simulink model "VFlexP"  (R2025a)
settings: Solver=ode23tb  StartTime=0.0  StopTime=40  FixedStep=5e-5
model workspace (MAT data in the model file):
  DCop_DCBUCK : object (value not decoded)
  Grid_CCVSC_idx = [2; 3; 4; 5; 6; 7; 8; 9; 10; 11; 12]
  Grid_CCVSCs = 1
  Grid_CCVSCs_buses = 1
  Grid_CCVSCs_toM = [0 1 0 0 0 0 0 0 0 0 0 0 ... (781 elements, 71x11)]
  Grid_C_Lines = [0.1 0.1 0.1 0.1]
  Grid_Cbuses = [0.05000002 0.10000002 0.10000002 0.10000002 0.05000002]
  Grid_DC : object (value not decoded)
  Grid_DCop_DCBUCK : object (value not decoded)
  Grid_DCop_DC_PES : object (value not decoded)
  Grid_DFIGs = 1
  Grid_DFIGs_buses = 1
  Grid_DGs : string (value not decoded)
  Grid_From_buses = [1 2 4 4]
  Grid_GFls = 1
  Grid_GFls_buses = 1
  Grid_GFr_idx = [1; 2; 3]
  Grid_GFrs = 1
  Grid_GFrs_buses = 1
  Grid_GFrs_toM = [1 0 0 0 0 0 0 0 0 1 0 0 ... (15 elements, 5x3)]
  Grid_IG_idx = 1
  Grid_IGs = 1
  Grid_IGs_buses = 1
  Grid_IGs_toM = [1; 0]
  Grid_L_Lines = [0.5 0.5 0.5 0.5]
  Grid_L_Loads = [0.000959999944704 0.000156249997559 0.00154855477548]
  Grid_Lines_fromM : object (value not decoded)
  Grid_Lines_toM : object (value not decoded)
  Grid_Load_buses = [2; 3; 4]
  Grid_Load_busesDC = []
  Grid_MGES_idx = [1; 2; 3]
  Grid_MGESs = 1
  Grid_MGESs_buses = [1; 5; 3]
  Grid_MGESs_toM = [1 0 0 0 0 0 0 0 0 1 0 0 ... (15 elements, 5x3)]
  Grid_MSGs = 1
  Grid_MSGs_buses = 1
  Grid_Nbuses = 5
  Grid_PQ_gen = [3; 2; 2]
  Grid_Ploads = [1250 4000 1250]
  Grid_PloadsDC = []
  Grid_Ps_lf = [0.274439537683 0.78 0.3]
  Grid_Qloads = [0.3 0.5 0.5]
  Grid_Qs_lf = [-0.0366071562958 0.126505596722 -0.0162964024532]
  Grid_R_Lines = [0.01 0.01 0.01 0.01]
  Grid_R_Loads = [3.9999997696 1.24999998047 3.8713869387]
  Grid_R_Loads_DC = 0
  Grid_Rcf = [50000000 50000000 50000000 50000000 50000000]
  Grid_SCs = 1
  Grid_SCs_buses = 1
  Grid_SG_idx = 1
  Grid_SGs = 1
  Grid_SGs_buses = 1
  Grid_SGs_toM = [1; 0]
  Grid_To_buses = [2 3 3 5]
  Grid_VCVSC_idx = [1; 2; 3; 4; 5; 6; 7; 8; 9; 10; 11; 12]
  Grid_VCVSCs = 1
  Grid_VCVSCs_buses = [1; 2; 3; 6; 8; 9; 12; 58; 59; 60; 63; 65]
  Grid_VCVSCs_toM = [1 0 0 0 0 0 0 0 0 0 0 0 ... (852 elements, 71x12)]
  Grid_VSM_idx = [1; 2; 3]
  Grid_VSMs = 1
  Grid_VSMs_buses = 1
  Grid_VSMs_toM = [1 0 0 0 0 0 0 0 0 1 0 0 ... (15 elements, 5x3)]
  Grid_admitt_matrix = [2.15353135314-19.7953135314i  -1.9801980198+19.801980198i; -1.9801980198+19.801980198i  2.15353135314-19.7953135314i]
  Grid_admitt_matrix_noloads = [1.98686468647-19.7953135314i  -1.9801980198+19.801980198i; -1.9801980198+19.801980198i  1.98686468647-19.7953135314i]
  Grid_bus = [1; 2; 6; 7; 8]
  Grid_busDC_complexity = [1 1 1]
  Grid_busDC_complexity_PF = [2 2 2]
  Grid_bus_complexity = [1 1 1 1 1]
  Grid_bus_complexity_PF = [1 1 1 1 1]
  Grid_buses_lf = [1; 5; 3]
  Grid_conductance_matrix = [100.00000002  -100  0; -100  200.00000002  -100; 0  -100  100.00000002]
  Grid_conductance_matrix_noloads = [100.00000002  -100  0; -100  200.00000002  -100; 0  -100  100.00000002]
  Grid_fref : object (value not decoded)
  Grid_gen_static_params : mBase (value not decoded)
  Grid_iPs_lf = [3.64378984326 1.28205128205 3.33333333333]
  Grid_iQs_lf = [-27.3170631425 7.90478860943 -61.3632366329]
  Grid_iadmitt_matrix = [2.88165849328-0.0982918688642i  2.87905051706-0.123273862303i; 2.87905051706-0.123273862303i  2.88165849328-0.0982918688642i]
  Grid_iadmitt_matrix_noloads = [37.5012524798-37.4874983544i  37.4987475202-37.5125016456i; 37.4987475202-37.5125016456i  37.5012524798-37.4874983544i]
  Grid_iconductance_matrix = [16666671.4556  16666671.4489  16666671.4456; 16666671.4489  16666671.4522  16666671.4489; 16666671.4456  16666671.4489  16666671.4556]
  Grid_iconductance_matrix_noloads = [16666671.4556  16666671.4489  16666671.4456; 16666671.4489  16666671.4522  16666671.4489; 16666671.4456  16666671.4489  16666671.4556]
  Grid_init_OK_bool = 1
  Grid_intconv_PF : object (value not decoded)
  Grid_lf_op : op_report (value not decoded)
  Grid_lineDC_complexity = [1 1]
  Grid_lineDC_complexity_PF = [2 2]
  Grid_line_complexity = [1 1 1 1]
  Grid_line_complexity_PF = [3 3 3 3]
  Grid_loadDC_complexity = []
  Grid_loadDC_complexity_PF = []
  Grid_load_complexity = [3 3 3]
  Grid_load_complexity_PF = [4 4 4]
  Grid_opDC_CCVSC : object (value not decoded)
  Grid_opDC_VSM : object (value not decoded)
  Grid_opGFr : object (value not decoded)
  Grid_opVCVSC : object (value not decoded)
  Grid_op_CCVSC : object (value not decoded)
  Grid_op_IG : object (value not decoded)
  Grid_op_MGES : object (value not decoded)
  Grid_op_SG : object (value not decoded)
  Grid_op_VSM : object (value not decoded)
  Grid_shift_lines = [0 0 0 0]
  Grid_tap_lines = [1 1 1 1]
  Grid_v_buses_mod = [1 1 1 0.9837920967 1]
  LinsysParamChangeStruct : Param1 (value not decoded)
  Lline = 0.01
  Rline = 1e-05
  linsys : object (value not decoded)
symbols that are objects in the model workspace (value not decoded): Grid_DCop_DC_PES, Grid_DCop_DCBUCK, Grid_op_CCVSC, Grid_op_IG, Grid_op_MGES, Grid_op_SG, Grid_op_VSM, Grid_opDC_CCVSC, Grid_opDC_VSM, Grid_opGFr, Grid_opVCVSC
undefined symbols (not defined in the file): block_buses_DC, block_idx, CCVSC_idx, Cf, costs, costs2, D, DFIGs_nodes, DiscIntNeverNeededParam, entity, Fb, Fi, From_nodes, grid_linsys, Grid_op_DFIG, Grid_op_DFIG_PQ, Grid_op_MSG, Grid_op_SC, Grid_op_VCVSC, H, initial_states_grid, K_1, K_3, K_5, K_A, K_C, K_IM, K_IR, K_P, K_PM, K_PR, K_S1, K_S2, K_S3, Ki_w, Kic, Kiv, Kp_id, Kp_theta, Kp_w, Kpc, Kpv, last_send, Lc, Lf, Lfd, Lkd1, Lkd2, Lkq1, Lkq2, Lkq3, Lmd, Lmq, Lsd, Lsq, m, M, Matrix_flux_to_i, mp, MSGs_buses ... (+44)
libraries: simulink x1048, eeGeneralControl x12
(part 7 of 50)

== system VFlexP/Grid/Generators/VSM ==
  note: port number 2
  note: do not rename this block, conditions to initialise the generator from PF result are set on this block's output
  note: port number 1
  elec_in : Inport
  v : Inport  Port=2
  AND : Logic  IconShape=distinctive  AllPortsSameDT=off  OutDataTypeStr=boolean
  AND1 : Logic  Inputs=3  IconShape=distinctive  AllPortsSameDT=off  OutDataTypeStr=boolean
  AND2 : Logic  IconShape=distinctive  AllPortsSameDT=off  OutDataTypeStr=boolean
  Abs{,1..3} (4 alike) : Abs  ZeroCross=off  SaturateOnIntegerOverflow=off
  Assignment : Assignment  NumberOfDimensions=2  DiagnosticForDimensions=Warning  IndexOptions=Assign all,Index vector (dialog)  Indices=1,block_idx  OutputSizes=1,1
  Atan2 : Trigonometry  Operator=atan2
  Cast To Boolean : DataTypeConversion  OutDataTypeStr=boolean  SaturateOnIntegerOverflow=off  RndMeth=Floor
  Cast To Double : DataTypeConversion  OutDataTypeStr=double  SaturateOnIntegerOverflow=off  RndMeth=Floor
  Cast To Double1 : DataTypeConversion  OutDataTypeStr=double  SaturateOnIntegerOverflow=off  RndMeth=Floor
  Cast To Double2 : DataTypeConversion  OutDataTypeStr=double  SaturateOnIntegerOverflow=off  RndMeth=Floor
  Compare To Constant : simulink/Logic and Bit Operations/Compare To Constant  relop=<=  const=0.001  OutDataTypeStr=boolean  ZeroCross=off
  Compare To Constant1 : simulink/Logic and Bit Operations/Compare To Constant  relop=<=  const=0.01  OutDataTypeStr=boolean  ZeroCross=off
  Compare To Constant2 : simulink/Logic and Bit Operations/Compare To Constant  relop=<=  const=0.2  OutDataTypeStr=boolean  ZeroCross=off
  Compare To Constant3 : simulink/Logic and Bit Operations/Compare To Constant  relop=>  const=4  OutDataTypeStr=boolean  ZeroCross=off
  Complex to Magnitude-Angle1 : ComplexToMagnitudeAngle  Output=Magnitude
  Complex to Real-Imag : ComplexToRealImag
  Conjugate : Math  Operator=conj  SignedPower=on  RndMeth=Zero
  Constant : Constant  Value=zeros(1, length(block_buses))  VectorParams1D=off
  Constant1 : Constant  Value=5*ones(1,length(block_idx))  VectorParams1D=off
  Constant2 : Constant  Value=zeros(1,length(block_idx))  VectorParams1D=off
  For Each Subsystem : Subsystem  TreatAsAtomicUnit=on
  Gain1 : Gain  Gain=-1
  Gain2 : Gain  Gain=-1
  Integrator : Integrator  ExternalReset=falling  InitialConditionSource=external  InitialCondition=[5]
  LPF1 : Subsystem
  LPF4 : Subsystem  Commented=through
  LPF5 : Subsystem  Commented=through
  Matrix Concatenate : Concatenate  NumInputs=6  Mode=Multidimensional array
  Matrix Concatenate1 : Concatenate  NumInputs=3  Mode=Multidimensional array
  Memory : Memory  InitialCondition=1
  Memory1 : Memory  InitialCondition=1
  Memory2 : Memory  InitialCondition=1
  NOT1 : Logic  Operator=NOT  IconShape=distinctive  AllPortsSameDT=off  OutDataTypeStr=boolean
  OR : Logic  Operator=OR  Inputs=3  IconShape=distinctive  AllPortsSameDT=off  OutDataTypeStr=boolean
  PC : Subsystem  mask(PC_VCVSC){Tf=Tf/(2*mp), mp=mp, nq=nq}
      mask prompts: Tf "Low-pass filter time constant (s)"; mp "Droop coefficient mp"; nq "Droop coefficient nq"
      mask help: Power controller of a grid-forming converter, including the droop control and low-pass filters for the power measurements.
      mask init: same as VFlexP/Grid/DCAC converters/DC_VCVSC/PC
  PI : Subsystem  Commented=on
  PI1 : Subsystem  Commented=on
  Product : Product
  Product1 : Product  OutDataTypeStr=double
  Product2 : Product  OutDataTypeStr=double
  Product3 : Product
  RL out : Subsystem  Variant=on  VariantControlMode=label  LabelModeActiveChoice=dynamic  mask{dynamic=Dynamic, R=R_out, L=L_out, fbase=50}
      mask prompts: dynamic "Dynamic behavior"; R "Series resistance (p.u.)"; L "Inductance (p.u.)"; fbase "Base frequency (Hz)"
      mask init: same as VFlexP/Grid/DCAC converters/DC_VCVSC/RL out
      mask TypeOptions dynamic: Static | Dynamic | Static omega
  Rate Limiter : RateLimiter  Commented=through  RisingSlewLimit=0.01  FallingSlewLimit=-0.01  SampleTimeMode=inherited
  Rate Limiter1 : RateLimiter  Commented=through  RisingSlewLimit=0.01  FallingSlewLimit=-0.01  SampleTimeMode=inherited
  Real-Imag to Complex : RealImagToComplex
  Real-Imag to Complex1 : RealImagToComplex
  Real-Imag to Complex3 : RealImagToComplex
  Reference frame transform1 : Subsystem
  Reference frame transform2 : Subsystem
  Reference frame transform3 : Subsystem
  Selector : Selector  NumberOfDimensions=2  InputPortWidth=3  IndexOptions=Index vector (dialog),Index vector (dialog)  Indices=1,block_idx  OutputSizes=1,1
  Selector1 : Selector  NumberOfDimensions=2  InputPortWidth=3  IndexOptions=Index vector (dialog),Index vector (dialog)  Indices=2,block_idx  OutputSizes=1,1
  Selector2 : Selector  NumberOfDimensions=2  InputPortWidth=3  IndexOptions=Index vector (dialog),Index vector (dialog)  Indices=3,block_idx  OutputSizes=1,1
  Selector3 : Selector  NumberOfDimensions=2  InputPortWidth=3  IndexOptions=Index vector (dialog),Index vector (dialog)  Indices=4,block_idx  OutputSizes=1,1
  Selector4 : Selector  NumberOfDimensions=2  InputPortWidth=3  IndexOptions=Index vector (dialog),Index vector (dialog)  Indices=5,block_idx  OutputSizes=1,1
  Selector5 : Selector  NumberOfDimensions=2  InputPortWidth=3  IndexOptions=Index vector (dialog),Index vector (dialog)  Indices=1,block_buses  OutputSizes=1,1
  Selector6 : Selector  NumberOfDimensions=2  InputPortWidth=3  IndexOptions=Index vector (dialog),Index vector (dialog)  Indices=2,block_buses  OutputSizes=1,1
  Selector7 : Selector  InputPortWidth=length(fref.ref_units)  IndexOptions=Index vector (dialog)  Indices=block_fref  OutputSizes=1
  Selector8 : Selector  InputPortWidth=length(fref.ref_units)  IndexOptions=Index vector (dialog)  Indices=block_fref  OutputSizes=1
  Signal Specification : SignalSpecification  Dimensions=[6 length(buses_lf)]
  Signal Specification1 : SignalSpecification  Dimensions=[3 length(block_buses)]
  Step : Step  Time=0.01  SampleTime=0  VectorParams1D=off  ZeroCross=off
  Sum10 : Sum  Inputs=|++
  Sum2 : Sum  Inputs=-+|
  Sum3 : Sum  Inputs=|+-
  Sum8 : Sum  Inputs=++|
  Sum9 : Sum  Inputs=|++
  Switch : Switch  Criteria=u2 > Threshold  SaturateOnIntegerOverflow=off  InputSameDT=off
  Switch1 : Switch  Criteria=u2 > Threshold  SaturateOnIntegerOverflow=off  InputSameDT=off
  Switch2 : Switch  Criteria=u2 > Threshold  SaturateOnIntegerOverflow=off  InputSameDT=off
  Terminator{,1..5} (6 alike) : Terminator
  VCC : Subsystem  Variant=on  VariantControlMode=label  LabelModeActiveChoice=static
  VI : Subsystem  mask{L=VI_L, R=VI_R, Tf=WOF_Tf}
      mask prompts: L "Inductance (pu)"; R "Resistance (pu)"; Tf "WOF time constant (s)"
      mask init: same as VFlexP/Grid/DCAC converters/DC_VCVSC/VI
  Zero : Constant  Value=0  OutDataTypeStr=Inherit: Inherit via back propagation
  Zero1 : Constant  Value=zeros(6, length(buses_lf))  VectorParams1D=off  OutDataTypeStr=Inherit: Inherit via back propagation
  connect : Subsystem
  frame : Integrator  InitialCondition=Grid_op_VSM.op.States(17).x'  IgnoreLimit=on
  trim_output : Subsystem
  vod : Sum  Inputs=++|
  elec_out : Outport
  i : Outport  Port=2
  wires:
  VCC/2(viqref) -> Reference frame transform3/3(in_q), [voq]
  VCC/1(vidref) -> Reference frame transform3/1(in_d), [vod]
  Memory1/1 -> Cast To Boolean/1
  Switch/1 -> Integrator/3
  Cast To Double2/1 -> Integrator/1
  AND1/1 -> Integrator/2, Cast To Double2/1
  [safe_to_connect] -> AND1/3
  Constant1/1 -> Switch/3
  Step/1 -> AND1/1, Switch/2
  Constant2/1 -> Switch/1
  Integrator/1 -> Compare To Constant3/1
  [connect] -> AND1/2
  AND2/1 -> Product2/1, Product1/1
  [connect] -> AND2/2
  [connected] -> NOT1/1
  NOT1/1 -> AND2/1
  [omega_to_follow] -> Sum10/2, Switch2/1
  Selector1/1 -> [P_s_to_follow]
  Memory/1 -> Cast To Double/1
  Selector5/1 -> trim_output/3(vd), [vdout]
  Selector6/1 -> trim_output/4(vq), [vqout]
  v/1 -> Selector5/1, Selector6/1
  trim_output/4(Out4) -> Terminator5/1
  trim_output/3(Out3) -> Terminator4/1
  trim_output/2(Out2) -> Terminator3/1
  trim_output/1(Out1) -> Terminator/1
  Zero1/1 -> Assignment/1
  [v_d_PCC] -> Real-Imag to Complex3/1
  [v_q_PCC] -> Real-Imag to Complex3/2
  Real-Imag to Complex3/1 -> Complex to Magnitude-Angle1/1
  [v_q_PCC] -> PC/5(voq)
  [v_d_PCC] -> PC/4(vodi)
  Signal Specification1/1 -> For Each Subsystem/1(In1)
  For Each Subsystem/1(Out1) -> i/1
  Constant/1 -> Matrix Concatenate1/3
  Matrix Concatenate1/1 -> Signal Specification1/1
  [vdout] -> Reference frame transform2/1(in_d), RL out/2(v_out_d)
  Reference frame transform2/2(out_q) -> [v_q_PCC]
  Reference frame transform2/1(out_d) -> [v_d_PCC]
  [vqout] -> RL out/4(v_out_q), Reference frame transform2/3(in_q)
  Memory2/1 -> [safe_to_connect]
  [connected] -> OR/3
  Compare To Constant2/1 -> OR/2
  OR/1 -> Memory2/1
  AND/1 -> OR/1
  Compare To Constant1/1 -> AND/1
  Abs3/1 -> Compare To Constant1/1
  Compare To Constant/1 -> AND/2
  Abs2/1 -> Compare To Constant/1
  Signal Specification/1 -> elec_out/1
  Abs1/1 -> Sum3/2, Compare To Constant2/1
  Cast To Boolean/1 -> [connect]
  Switch2/1 -> Rate Limiter/1
  PI1/1(Out1) -> Sum10/1
  Atan2/1 -> Product2/2, Abs3/1
  Product2/1 -> PI1/1(In1)
  Product1/1 -> PI/1(In1)
  PI/1(Out1) -> Sum9/1
  Sum3/1 -> Product1/2, Abs2/1
  Abs/1 -> Sum3/1
  Complex to Real-Imag/1 -> Atan2/2
  Complex to Real-Imag/2 -> Atan2/1
  Product/1 -> Complex to Real-Imag/1
  Conjugate/1 -> Product/2
  Real-Imag to Complex/1 -> Product/1, Abs/1
  Real-Imag to Complex1/1 -> Conjugate/1, Abs1/1
  [voq] -> Real-Imag to Complex1/2
  [vod] -> Real-Imag to Complex1/1
  [v_q_PCC] -> Real-Imag to Complex/2
  [v_d_PCC] -> Real-Imag to Complex/1
  Cast To Double1/1 -> Matrix Concatenate/5
  Cast To Double/1 -> Matrix Concatenate/6
  Selector4/1 -> Memory1/1
  [connected] -> Memory/1
  [connect] -> Cast To Double1/1
  Assignment/1 -> Signal Specification/1
  elec_in/1 -> Selector/1, Selector1/1, Selector2/1, Selector3/1, Selector4/1
  Matrix Concatenate/1 -> Assignment/2
  [omega] -> Matrix Concatenate/1  "omega"
  Complex to Magnitude-Angle1/1 -> LPF1/1(In1)  "v"
  [P_s] -> Matrix Concatenate/2  "P_s"
  [Q_s] -> Matrix Concatenate/4
  Selector2/1 -> [v_to_follow]
  Selector/1 -> [omega_to_follow]
  Selector3/1 -> [Q_s_to_follow]
  RL out/4(v_outq) -> Terminator2/1
  RL out/3(v_outd) -> Terminator1/1
  connect/2(iq_real) -> Reference frame transform1/3(in_q), Matrix Concatenate1/2, trim_output/2(iq)
  connect/1(id_real) -> Reference frame transform1/1(in_d), Matrix Concatenate1/1, trim_output/1(id)
  VI/2(vq) -> Sum8/1
  VI/1(vd) -> vod/1
  Reference frame transform1/1(out_d) -> [iod]
  RL out/2(iq) -> connect/2(iq)
  Reference frame transform3/2(out_q) -> RL out/3(v_in_q)
  Reference frame transform3/1(out_d) -> RL out/1(v_in_d)
  Reference frame transform1/2(out_q) -> [ioq]
  [ioq] -> PC/1(ioq)
  [iod] -> PC/2(iodi)
  PC/2(Out2) -> [vodref]
  PC/1(omega) -> [omega]
  [theta] -> Reference frame transform3/2(theta)
  [omega] -> VCC/5(omega)
  [vodref] -> vod/2
  Zero/1 -> Sum8/2
  [iod] -> VCC/3(iod)
  [ioq] -> VCC/4(ioq)
  Gain1/1 -> Reference frame transform1/2(theta)
  [theta] -> Gain1/1
  RL out/1(id) -> connect/1(id)
  Sum2/1 -> Product3/1
  [omega_ref] -> Selector7/1  "ref_omega"
  [omega] -> Sum2/2  "omega"
  connect/3(connected) -> [connected]
  PC/3(P_f) -> [P_f], [P_s]
  PC/4(Q_f) -> [Q_f], [Q_s]
  [P_s_to_follow] -> PC/7(Psp)
  frame/1 -> [theta]
  Product3/1 -> frame/1
  Rate Limiter1/1 -> LPF5/1(In1)
  [theta] -> Gain2/1
  Gain2/1 -> Reference frame transform2/2(theta)
  [iod] -> VI/1(id)
  [ioq] -> VI/2(iq)
  [omega] -> VI/3(omega)
  vod/1 -> VCC/1(vodref)
  Sum8/1 -> VCC/2(voqref)
  Rate Limiter/1 -> LPF4/1(In1)
  Sum10/1 -> Switch2/3
  Sum9/1 -> Switch1/3
  [connected] -> Switch1/2, Switch2/2
  Switch1/1 -> Rate Limiter1/1
  [v_to_follow] -> Sum9/2, Switch1/1
  LPF4/1(Out1) -> PC/6(omegasp)
  LPF5/1(Out1) -> PC/3(Eref)
  Selector7/1 -> Sum2/1
  [omega_base] -> Selector8/1
  Selector8/1 -> Product3/2
  LPF1/1(Out1) -> Matrix Concatenate/3
  Compare To Constant3/1 -> connect/3(connect)

== system VFlexP/Grid/Generators_DC/DCBUCK ==
  v : Inport
  ref : Inport  Port=2
  Constant2 : Constant  Value=block_Pg./(DC.v(block_buses)*Sb)  VectorParams1D=off
  Gain : Gain  Gain=0.6
  Gain1 : Gain  Gain=565.4867
  Gain4 : Gain  Gain=1/1.5915e-04
  Gain5 : Gain  Gain=0.01
  Integrator : Integrator  InitialCondition=Grid_DCop_DCBUCK.op.States(1).x'
  Integrator1 : Integrator  InitialCondition=Grid_DCop_DCBUCK.op.States(2).x'
  Selector : Selector  InputPortWidth=DC.Nbuses  IndexOptions=Index vector (dialog)  Indices=block_buses  OutputSizes=1
  Selector1 : Selector  Commented=on  InputPortWidth=3  IndexOptions=Index vector (dialog)  Indices=[1 3]  OutputSizes=1
  State-Space : StateSpace  A=[]  B=[]  C=[]  D=block_toM  InitialCondition=0  ParameterTunability=Optimized
  Sum : Sum  Inputs=|++
  Sum2 : Sum  Inputs=|+-
  Sum3 : Sum  Inputs=++-
  Transpose : Math  Operator=transpose
  Transpose1 : Math  Operator=transpose
  i : Outport
  wires:
  Gain5/1 -> Sum3/3
  Selector/1 -> Sum3/1
  v/1 -> Selector/1
  ref/1 -> Selector1/1
  Constant2/1 -> Sum2/1
  Sum3/1 -> Gain4/1
  Transpose1/1 -> i/1
  Sum2/1 -> Gain/1, Gain1/1
  Gain4/1 -> Integrator/1
  Integrator1/1 -> Sum/1
  Gain/1 -> Sum/2
  Sum/1 -> Sum3/2
  Gain1/1 -> Integrator1/1
  Transpose/1 -> State-Space/1
  Integrator/1 -> Transpose/1, Gain5/1, Sum2/2
  State-Space/1 -> Transpose1/1

== system VFlexP/Grid/Generators_DC/DC_PES ==
  v : Inport
  ref : Inport  Port=2
  Gain : Gain
  Gain1 : Gain  Gain=5.4131
  Gain2 : Gain  Gain=0.0018
  Gain3 : Gain  Gain=5.0000
  Integrator : Integrator  InitialCondition=Grid_DCop_DC_PES.op.States(1).x'
  Integrator1 : Integrator  InitialCondition=Grid_DCop_DC_PES.op.States(2).x'
  Integrator2 : Integrator  InitialCondition=Grid_DCop_DC_PES.op.States(3).x'
  One : Constant  Value=DC.v(block_buses)  OutDataTypeStr=Inherit: Inherit via back propagation
  Selector : Selector  InputPortWidth=DC.Nbuses  IndexOptions=Index vector (dialog)  Indices=block_buses  OutputSizes=1
  Selector1 : Selector  Commented=on  InputPortWidth=3  IndexOptions=Index vector (dialog)  Indices=[1 3]  OutputSizes=1
  Square : Math  Operator=square
  State-Space : StateSpace  A=[]  B=[]  C=[]  D=block_toM  InitialCondition=0  ParameterTunability=Optimized
  Step2 : Step  Time=0.1  After=0.1  SampleTime=0
  Sum : Sum  Inputs=+|+|+
  Sum1 : Sum  Inputs=|+-
  Sum13 : Sum  Inputs=|++
  Sum2 : Sum  Inputs=|+-
  Sum3 : Sum  Inputs=|+-
  Transpose : Math  Operator=transpose
  Transpose1 : Math  Operator=transpose
  WOF_d : Subsystem
  i : Outport
  wires:
  State-Space/1 -> Transpose1/1
  Transpose/1 -> State-Space/1
  Transpose1/1 -> i/1
  Sum3/1 -> Gain2/1, Gain1/1, Gain3/1
  ref/1 -> Selector1/1
  v/1 -> Selector/1
  Selector/1 -> Square/1
  One/1 -> Sum3/1
  Sum1/1 -> Gain/1
  Integrator1/1 -> Sum1/2, Transpose/1
  Gain/1 -> Integrator1/1
  Sum2/1 -> Sum1/1
  Gain2/1 -> WOF_d/1(In1)
  Sum13/1 -> Sum2/1
  Integrator2/1 -> Sum13/2
  Sum/1 -> Sum13/1
  Gain3/1 -> Integrator/1
  Square/1 -> Sum3/2
  Gain1/1 -> Sum/1
  Integrator/1 -> Sum/3
  WOF_d/1(Out1) -> Sum/2

== system VFlexP/Grid/Grid/Dynamic ==
  i_from_gen : Inport
  Buses : Subsystem
  Goto Tag Visibility : GotoTagVisibility  GotoTag=Cbuses
  Lines : Subsystem
  Lines to buses : Subsystem
  Loads : Subsystem
  Loads to buses : Subsystem
  Selector2 : Selector  NumberOfDimensions=2  InputPortWidth=Nnodes  IndexOptions=Select all,Index vector (dialog)  Indices=1,Load_buses  OutputSizes=1,1
  Selector4 : Selector  NumberOfDimensions=2  InputPortWidth=Nnodes  IndexOptions=Select all,Index vector (dialog)  Indices=From_nodes,From_buses  OutputSizes=1,1
  Selector6 : Selector  NumberOfDimensions=2  InputPortWidth=Nnodes  IndexOptions=Select all,Index vector (dialog)  Indices=To_nodes,To_buses  OutputSizes=1,1
  Step : Step  Before=ones(1, length(From_buses))  After=[1 ones(1, length(From_buses)-1)]  SampleTime=0
  Sum : Sum  Inputs=++|
  Sum1 : Sum  Inputs=|++
  connect : Subsystem
  iCbuses : Subsystem
  iP : Subsystem
  v_buses : Outport
  tag scope: Cbuses=scoped
  wires:
  Buses/1(v) -> [v_buses], v_buses/1  "v"
  [i_from_lines] -> Sum/2
  [i_to_loads] -> Sum1/1
  Lines to buses/2(i_out_buses) -> [i_to_lines]
  Loads to buses/1(i_out_buses) -> [i_to_loads]
  iP/1(Out1) -> Loads/3(iP)
  Selector6/1 -> Lines/2(v_out)
  [v_buses] -> Selector2/1
  connect/1(Out1) -> Loads/2(connected)
  [v_buses] -> Selector6/1
  Loads/1(i) -> Loads to buses/1(i_loads)
  Sum/1 -> Buses/1(i_in)
  Selector4/1 -> Lines/1(v_in)
  Selector2/1 -> Loads/1(v_in)
  [v_buses] -> Selector4/1
  [i_to_lines] -> Sum1/2
  Step/1 -> iCbuses/1(In1), Lines/3(connected)
  i_from_gen/1 -> Sum/1
  Sum1/1 -> Buses/2(i_out)
  Lines to buses/1(i_in_buses) -> [i_from_lines]
  Lines/1(i) -> Lines to buses/1(i)
  iCbuses/1(Out1) -> [Cbuses]

== system VFlexP/Grid/Grid/Static ==
  i_from_gen : Inport
  Complex to Real-Imag : ComplexToRealImag
  Constant : Constant  Value=zeros(1, Nbuses)  VectorParams1D=off
  Gain : Gain  Gain=iadmitt_matrix  Multiplication=Matrix(K*u)
  Matrix Concatenate : Concatenate  NumInputs=3  Mode=Multidimensional array
  Real-Imag to Complex : RealImagToComplex
  Scope : Scope
      settings: ActiveDisplayYMinimum=1.0463  ActiveDisplayYMaximum=1.1306
  Selector : Selector  NumberOfDimensions=2  InputPortWidth=3  IndexOptions=Index vector (dialog),Select all  Indices=1,find(bus_complexity == 1)  OutputSizes=1,1
  Selector1 : Selector  NumberOfDimensions=2  InputPortWidth=3  IndexOptions=Index vector (dialog),Select all  Indices=2,find(bus_complexity == 1)  OutputSizes=1,1
  Transpose : Math  Operator=transpose
  Transpose2 : Math  Operator=transpose
  v_buses : Outport
  wires:
  Constant/1 -> Matrix Concatenate/3
  Selector/1 -> Real-Imag to Complex/1  "id1"
  Selector1/1 -> Real-Imag to Complex/2  "iq1"
  i_from_gen/1 -> Selector1/1, Selector/1
  Real-Imag to Complex/1 -> Transpose/1
  Complex to Real-Imag/1 -> Matrix Concatenate/1, Scope/1
  Complex to Real-Imag/2 -> Matrix Concatenate/2
  Transpose2/1 -> Complex to Real-Imag/1
  Transpose/1 -> Gain/1
  Gain/1 -> Transpose2/1
  Matrix Concatenate/1 -> v_buses/1

== system VFlexP/Grid/Grid_DC/dynamic ==
  i_from_gen_dc : Inport
  BusesDC : Subsystem
  DC_Lines_toM1 : Subsystem  TreatAsAtomicUnit=on
  DClines : Subsystem
  Loads : Subsystem  Commented=on
  Loads to buses : Subsystem  Commented=on
  One1 : Constant  Commented=on  Value=ones(1, length(R_Loads_DC))  VectorParams1D=off  OutDataTypeStr=Inherit: Inherit via back propagation
  Scope : Scope
      settings: ActiveDisplayYMinimum=-0.01246  ActiveDisplayYMaximum=0.11218
  Selector2 : Selector  NumberOfDimensions=2  InputPortWidth=Nnodes  IndexOptions=Select all,Index vector (dialog)  Indices=From_nodes,DC.to  OutputSizes=1,1
  Selector4 : Selector  NumberOfDimensions=2  InputPortWidth=Nnodes  IndexOptions=Select all,Index vector (dialog)  Indices=From_nodes,DC.from  OutputSizes=1,1
  Selector5 : Selector  Commented=on  NumberOfDimensions=2  InputPortWidth=Nnodes  IndexOptions=Select all,Index vector (dialog)  Indices=1,Load_busesDC  OutputSizes=1,1
  Step1 : Step  Commented=on  Time=1.2  Before=zeros(1, DC.Nbuses)  After=[-0.01 zeros(1, DC.Nbuses-1)]  SampleTime=0  VectorParams1D=off
  Step3 : Step  Commented=on  Before=zeros(1, DC.Nbuses)  After=[0.01 zeros(1, DC.Nbuses-1)]  SampleTime=0  VectorParams1D=off
  Sum : Sum  Commented=on  Inputs=|++
  Sum6 : Sum  Inputs=|++
  Sum7 : Sum  Inputs=|++
  Sum8 : Sum  Inputs=|++
  v_buses_dc : Outport
  wires:
  BusesDC/1(v) -> v_buses_dc/1, [v_buses]
  [v_buses] -> Selector2/1
  Selector2/1 -> DClines/2(V_dc_out)
  Sum6/1 -> BusesDC/1(Input)
  Selector4/1 -> DClines/1(V_dc_In)
  Loads/1(i) -> Loads to buses/1(i_loads)
  Selector5/1 -> Loads/1(v_in)
  i_from_gen_dc/1 -> Sum6/2
  Sum8/1 -> BusesDC/2(Input1)
  Sum7/1 -> Sum8/1
  DC_Lines_toM1/1(i_from_lines) -> Sum6/1
  [v_buses] -> Selector4/1
  [i_to_loadsDC] -> Sum8/2
  DClines/1(i) -> DC_Lines_toM1/1(i)
  One1/1 -> Loads/2(connected)
  DC_Lines_toM1/2(i_to_lines) -> Sum7/1
  Loads to buses/1(i_out_buses) -> Scope/1, [i_to_loadsDC]
  [v_buses] -> Selector5/1
  Step3/1 -> Sum/1
  Sum/1 -> Sum7/2
  Step1/1 -> Sum/2

== system VFlexP/Grid/Grid_DC/static ==
  i_from_gen_dc : Inport
  Gain : Gain  Gain=iconductance_matrix  Multiplication=Matrix(K*u)
  LPF_d1 : Subsystem
  Transpose : Math  Operator=transpose
  Transpose1 : Math  Operator=transpose
  v_buses_dc : Outport
  wires:
  Gain/1 -> Transpose1/1
  LPF_d1/1(v_buses_dc) -> v_buses_dc/1
  Transpose1/1 -> LPF_d1/1(In1)
  Transpose/1 -> Gain/1
  i_from_gen_dc/1 -> Transpose/1

== system VFlexP/Grid/Secondary Control/MAS messages ==
  tertiary_refs : Inport
  Constant1 : Constant  Value=1000*ones(1, length(buses_lf))  VectorParams1D=off
  Constant2 : Constant  Value=100*ones(1, length(buses_lf))  VectorParams1D=off
  Costs : RandomNumber  Mean=2*ones(1,length(buses_lf))  Variance=1*ones(1,length(buses_lf))  Seed=1:length(buses_lf)  SampleTime=100  VectorParams1D=off
  Goto Tag Visibility : GotoTagVisibility  GotoTag=Pmax
  Goto Tag Visibility1 : GotoTagVisibility  GotoTag=Snom
  Goto Tag Visibility2 : GotoTagVisibility  GotoTag=costs
  ID1 : Subsystem  VariantControl=multi-agent  mask(gen_agent){ID=1, Leader=Leader, NeighN=2, Neigh1=5, Neigh2=2, Neigh3=0, Neigh4=0, Neigh5=0}
      mask prompts: ID "ID number"; Leader "Leader multi-agent"; NeighN "Number of neighbors"; Neigh1 "Neighbor 1"; Neigh2 "Neighbor 2"; Neigh3 "Neighbor 3"; Neigh4 "Neighbor 4"; Neigh5 "Neighbor 5"
      mask init:
      | block = gcb;
      | NeighN_value = str2double(NeighN);
      | bvarname = get_param(strcat(bdroot, "/", ...
      |     string(extractBetween(gcb, [bdroot '/'], '/'))), 'bvarname');
      | set_param([block '/sentToWorkspace'], 'VariableName', ['sent_' bvarname 'ID' ID])
      | set_param([block '/followingToWorkspace'], 'VariableName', ['following_' bvarname 'ID' ID])
      | set_param([block '/sendingToWorkspace'], 'VariableName', ['sending_' bvarname 'ID' ID])
      | set_param([block '/Receive'], 'MulticastTag', ...
      |     ['ID' ID])
      | set_param([block '/ID'], 'Value', ID)
      | IDnumber = str2double(ID);
      | if strcmp(Leader, "Leader")
      |     set_param([block '/Leader'], 'Value', '1')
      | else
      |     set_param([block '/Leader'], 'Value', '0')
      | end
      | bl_send = find_system(gcb, 'MatchFilter', @Simulink.match.allVariants, 'LookUnderMasks', 'on','MaskType','Send_to_neighbor');
      | 
      | set_param([block '/neigh_left'], 'Value', NeighN)
      | switch NeighN_value % Neighbors
      |     case 1
      |         for i=1:length(bl_send)
      |             set_param(bl_send{i}, 'LabelModeActiveChoice', 'one')
      |             set_param([bl_send{i} '/one/select/Neighbor'], 'const', Neigh1)
      |             set_param([bl_send{i} '/one/Cast'], 'MulticastTag', ['ID' Neigh1])
      |             set_param([bl_send{i} '/one/Castall'], 'MulticastTag', ['ID' Neigh1])
      |         end
      |     case 2
      |         for i=1:length(bl_send)
      |             set_param(bl_send{i}, 'LabelModeActiveChoice', 'two')
      |             set_param([bl_send{i} '/two/select/Neighbor1'], 'const', Neigh1)
      |             set_param([bl_send{i} '/two/Cast1'], 'MulticastTag', ['ID' Neigh1])
      |             set_param([bl_send{i} '/two/Cast1all'], 'MulticastTag', ['ID' Neigh1])
      |             set_param([bl_send{i} '/two/select/Neighbor2'], 'const', Neigh2)
      |             set_param([bl_send{i} '/two/Cast2'], 'MulticastTag', ['ID' Neigh2])
      |             set_param([bl_send{i} '/two/Cast2all'], 'MulticastTag', ['ID' Neigh2])
      |         end
      |     case 3
      |         for i=1:length(bl_send)
      |             set_param(bl_send{i}, 'LabelModeActiveChoice', 'three')
      |             set_param([bl_send{i} '/three/select/Neighbor1'], 'const', Neigh1)
      |             set_param([bl_send{i} '/three/Cast1'], 'MulticastTag', ['ID' Neigh1])
      |             set_param([bl_send{i} '/three/Cast1all'], 'MulticastTag', ['ID' Neigh1])
      |             set_param([bl_send{i} '/three/select/Neighbor2'], 'const', Neigh2)
      |             set_param([bl_send{i} '/three/Cast2'], 'MulticastTag', ['ID' Neigh2])
      |             set_param([bl_send{i} '/three/Cast2all'], 'MulticastTag', ['ID' Neigh2])
      |             set_param([bl_send{i} '/three/select/Neighbor3'], 'const', Neigh3)
      |             set_param([bl_send{i} '/three/Cast3'], 'MulticastTag', ['ID' Neigh3])
      |             set_param([bl_send{i} '/three/Cast3all'], 'MulticastTag', ['ID' Neigh3])
      |         end
      |     case 4
      |         for i=1:length(bl_send)
      |             set_param(bl_send{i}, 'LabelModeActiveChoice', 'four')
      |             set_param([bl_send{i} '/four/select/Neighbor1'], 'const', Neigh1)
      |             set_param([bl_send{i} '/four/Cast1'], 'MulticastTag', ['ID' Neigh1])
      |             set_param([bl_send{i} '/four/Cast1all'], 'MulticastTag', ['ID' Neigh1])
      |             set_param([bl_send{i} '/four/select/Neighbor2'], 'const', Neigh2)
      |             set_param([bl_send{i} '/four/Cast2'], 'MulticastTag', ['ID' Neigh2])
      |             set_param([bl_send{i} '/four/Cast2all'], 'MulticastTag', ['ID' Neigh2])
      |             set_param([bl_send{i} '/four/select/Neighbor3'], 'const', Neigh3)
      |             set_param([bl_send{i} '/four/Cast3'], 'MulticastTag', ['ID' Neigh3])
      |             set_param([bl_send{i} '/four/Cast3all'], 'MulticastTag', ['ID' Neigh3])
      |             set_param([bl_send{i} '/four/select/Neighbor4'], 'const', Neigh4)
      |             set_param([bl_send{i} '/four/Cast4'], 'MulticastTag', ['ID' Neigh4])
      |             set_param([bl_send{i} '/four/Cast4all'], 'MulticastTag', ['ID' Neigh4])
      |         end
      |     case 5
      |         for i=1:length(bl_send)
      |             set_param(bl_send{i}, 'LabelModeActiveChoice', 'five')
      |             set_param([bl_send{i} '/five/select/Neighbor1'], 'const', Neigh1)
      |             set_param([bl_send{i} '/five/Cast1'], 'MulticastTag', ['ID' Neigh1])
      |             set_param([bl_send{i} '/five/Cast1all'], 'MulticastTag', ['ID' Neigh1])
      |             set_param([bl_send{i} '/five/select/Neighbor2'], 'const', Neigh2)
      |             set_param([bl_send{i} '/five/Cast2'], 'MulticastTag', ['ID' Neigh2])
      |             set_param([bl_send{i} '/five/Cast2all'], 'MulticastTag', ['ID' Neigh2])
      |             set_param([bl_send{i} '/five/select/Neighbor3'], 'const', Neigh3)
      |             set_param([bl_send{i} '/five/Cast3'], 'MulticastTag', ['ID' Neigh3])
      |             set_param([bl_send{i} '/five/Cast3all'], 'MulticastTag', ['ID' Neigh3])
      |             set_param([bl_send{i} '/five/select/Neighbor4'], 'const', Neigh4)
      |             set_param([bl_send{i} '/five/Cast4'], 'MulticastTag', ['ID' Neigh4])
      |             set_param([bl_send{i} '/five/Cast4all'], 'MulticastTag', ['ID' Neigh4])
      |             set_param([bl_send{i} '/five/select/Neighbor5'], 'const', Neigh5)
      |             set_param([bl_send{i} '/five/Cast5'], 'MulticastTag', ['ID' Neigh5])
      |             set_param([bl_send{i} '/five/Cast5all'], 'MulticastTag', ['ID' Neigh5])
      |         end
      | end
      mask TypeOptions Leader: No leader | Leader
      mask TypeOptions NeighN: 1 | 2 | 3 | 4 | 5
      mask Callback NeighN:
      | block = gcb;
      | NeighN = str2double(get_param(block, 'NeighN'));
      | param_vis = get_param(block,'MaskVisibilities');
      | block_params = string(fieldnames(get_param(block, 'DialogParameters')));
      | param_vis(find(block_params == 'Neigh1'):find(block_params == 'Neigh5')) = cellstr("on");
      | if NeighN < 5 % Hide some
      |     param_vis(find(block_params == 'Neigh1')+NeighN:find(block_params == 'Neigh5')) = cellstr("off");
      | end
      | set_param(block,'MaskVisibilities',param_vis)
      mask DialogControl Container8 Prompt: Parameters
  ID2 : Subsystem  VariantControl=multi-agent  mask(gen_agent){ID=2, Leader=No leader, NeighN=2, Neigh1=1, Neigh2=3, Neigh3=0, Neigh4=0, Neigh5=0}
      mask prompts: ID "ID number"; Leader "Leader multi-agent"; NeighN "Number of neighbors"; Neigh1 "Neighbor 1"; Neigh2 "Neighbor 2"; Neigh3 "Neighbor 3"; Neigh4 "Neighbor 4"; Neigh5 "Neighbor 5"
      mask init: same as VFlexP/Grid/Secondary Control/MAS messages/ID1
      mask TypeOptions Leader: No leader | Leader
      mask TypeOptions NeighN: 1 | 2 | 3 | 4 | 5
      mask Callback NeighN:
      | block = gcb;
      | NeighN = str2double(get_param(block, 'NeighN'));
      | param_vis = get_param(block,'MaskVisibilities');
      | block_params = string(fieldnames(get_param(block, 'DialogParameters')));
      | param_vis(find(block_params == 'Neigh1'):find(block_params == 'Neigh5')) = cellstr("on");
      | if NeighN < 5 % Hide some
      |     param_vis(find(block_params == 'Neigh1')+NeighN:find(block_params == 'Neigh5')) = cellstr("off");
      | end
      | set_param(block,'MaskVisibilities',param_vis)
      mask DialogControl Container8 Prompt: Parameters
  ID3 : Subsystem  VariantControl=multi-agent  mask(gen_agent){ID=3, Leader=No leader, NeighN=2, Neigh1=2, Neigh2=4, Neigh3=0, Neigh4=0, Neigh5=0}
      mask prompts: ID "ID number"; Leader "Leader multi-agent"; NeighN "Number of neighbors"; Neigh1 "Neighbor 1"; Neigh2 "Neighbor 2"; Neigh3 "Neighbor 3"; Neigh4 "Neighbor 4"; Neigh5 "Neighbor 5"
      mask init: same as VFlexP/Grid/Secondary Control/MAS messages/ID1
      mask TypeOptions Leader: No leader | Leader
      mask TypeOptions NeighN: 1 | 2 | 3 | 4 | 5
      mask Callback NeighN:
      | block = gcb;
      | NeighN = str2double(get_param(block, 'NeighN'));
      | param_vis = get_param(block,'MaskVisibilities');
      | block_params = string(fieldnames(get_param(block, 'DialogParameters')));
      | param_vis(find(block_params == 'Neigh1'):find(block_params == 'Neigh5')) = cellstr("on");
      | if NeighN < 5 % Hide some
      |     param_vis(find(block_params == 'Neigh1')+NeighN:find(block_params == 'Neigh5')) = cellstr("off");
      | end
      | set_param(block,'MaskVisibilities',param_vis)
      mask DialogControl Container8 Prompt: Parameters
  ID4 : Subsystem  VariantControl=multi-agent  mask(gen_agent){ID=4, Leader=No leader, NeighN=2, Neigh1=3, Neigh2=5, Neigh3=0, Neigh4=0, Neigh5=0}
      mask prompts: ID "ID number"; Leader "Leader multi-agent"; NeighN "Number of neighbors"; Neigh1 "Neighbor 1"; Neigh2 "Neighbor 2"; Neigh3 "Neighbor 3"; Neigh4 "Neighbor 4"; Neigh5 "Neighbor 5"
      mask init: same as VFlexP/Grid/Secondary Control/MAS messages/ID1
      mask TypeOptions Leader: No leader | Leader
      mask TypeOptions NeighN: 1 | 2 | 3 | 4 | 5
      mask Callback NeighN:
      | block = gcb;
      | NeighN = str2double(get_param(block, 'NeighN'));
      | param_vis = get_param(block,'MaskVisibilities');
      | block_params = string(fieldnames(get_param(block, 'DialogParameters')));
      | param_vis(find(block_params == 'Neigh1'):find(block_params == 'Neigh5')) = cellstr("on");
      | if NeighN < 5 % Hide some
      |     param_vis(find(block_params == 'Neigh1')+NeighN:find(block_params == 'Neigh5')) = cellstr("off");
      | end
      | set_param(block,'MaskVisibilities',param_vis)
      mask DialogControl Container8 Prompt: Parameters
  ID5 : Subsystem  VariantControl=multi-agent  mask(gen_agent){ID=5, Leader=No leader, NeighN=2, Neigh1=4, Neigh2=1, Neigh3=0, Neigh4=0, Neigh5=0}
      mask prompts: ID "ID number"; Leader "Leader multi-agent"; NeighN "Number of neighbors"; Neigh1 "Neighbor 1"; Neigh2 "Neighbor 2"; Neigh3 "Neighbor 3"; Neigh4 "Neighbor 4"; Neigh5 "Neighbor 5"
      mask init: same as VFlexP/Grid/Secondary Control/MAS messages/ID1
      mask TypeOptions Leader: No leader | Leader
      mask TypeOptions NeighN: 1 | 2 | 3 | 4 | 5
      mask Callback NeighN:
      | block = gcb;
      | NeighN = str2double(get_param(block, 'NeighN'));
      | param_vis = get_param(block,'MaskVisibilities');
      | block_params = string(fieldnames(get_param(block, 'DialogParameters')));
      | param_vis(find(block_params == 'Neigh1'):find(block_params == 'Neigh5')) = cellstr("on");
      | if NeighN < 5 % Hide some
      |     param_vis(find(block_params == 'Neigh1')+NeighN:find(block_params == 'Neigh5')) = cellstr("off");
      | end
      | set_param(block,'MaskVisibilities',param_vis)
      mask DialogControl Container8 Prompt: Parameters
  Scope : Scope
      settings: ActiveDisplayYMinimum=3.7204  ActiveDisplayYMaximum=6.2533  DataLoggingVariableName=ScopeData2
  Scope1 : Scope
      settings: ActiveDisplayYMinimum=0.24945  ActiveDisplayYMaximum=4.0188
  Scope2 : Scope  NumInputPorts=2
      settings: ActiveDisplayYMinimum=9.9395  ActiveDisplayYMaximum=10.281  DataLoggingVariableName=ScopeData3
  Selector : Selector  NumberOfDimensions=2  InputPortWidth=3  IndexOptions=Index vector (dialog),Select all  Indices=1:6,1  OutputSizes=1,1
  Selector1 : Selector  NumberOfDimensions=2  InputPortWidth=3  IndexOptions=Index vector (dialog),Select all  Indices=7,1  OutputSizes=1,1
  Selector2 : Selector  NumberOfDimensions=2  InputPortWidth=3  IndexOptions=Index vector (dialog),Select all  Indices=8,1  OutputSizes=1,1
  Selector3 : Selector  NumberOfDimensions=2  InputPortWidth=3  IndexOptions=Index vector (dialog),Select all  Indices=2,1  OutputSizes=1,1
  Sum of Elements : Sum  Inputs=+
  Sum of Elements1 : Sum  Inputs=+
  concat : Concatenate  NumInputs=length(buses_lf)  Mode=Multidimensional array  ConcatenateDimension=2
  secondary_refs : Outport
  tag scope: Pmax=scoped, Snom=scoped, costs=scoped
  wires:
  concat/1 -> Selector2/1, Selector1/1, Selector/1
  tertiary_refs/1 -> Selector3/1, ID1/1(in), ID2/1(in), ID3/1(in), ID4/1(in), ID5/1(in)
  Constant2/1 -> [Pmax]
  Constant1/1 -> [Snom]
  ID1/1(out) -> concat/1
  Selector/1 -> secondary_refs/1
  Selector1/1 -> Sum of Elements1/1, Scope/1
  Selector2/1 -> Scope1/1
  Selector3/1 -> Sum of Elements/1
  Sum of Elements/1 -> Scope2/1
  Sum of Elements1/1 -> Scope2/2
  Costs/1 -> [costs]
  ID2/1(out) -> concat/2
  ID3/1(out) -> concat/3
  ID4/1(out) -> concat/4
  ID5/1(out) -> concat/5

== system VFlexP/Grid/Secondary Control/Matrices ==
  tertiary_refs : Inport
  start_SC : Inport  Port=2
  elec : Inport  Port=3
  Gain : Gain  Gain=A_f_sc  Multiplication=Matrix(K*u)
  Gain1 : Gain  Gain=g_f_sc'
  Gain10 : Gain  Gain=[sum(A_f_sc, 2)'; sum(A_P_sc, 2)'; sum(A_v_sc, 2)'; sum(A_Q_sc, 2)']
  Gain2 : Gain  Gain=A_P_sc  Multiplication=Matrix(K*u)
  Gain3 : Gain  Gain=g_P_sc'
  Gain4 : Gain  Gain=A_v_sc  Multiplication=Matrix(K*u)
  Gain5 : Gain  Gain=g_v_sc'
  Gain6 : Gain  Gain=g_Q_sc'
  Gain7 : Gain  Gain=A_Q_sc  Multiplication=Matrix(K*u)
  Gain8 : Gain  Gain=repmat([1 0.01 1 0.01]', 1, length(buses_lf))
  Gain9 : Gain  Gain=-1
  Integrator : Integrator
  Matrix Concatenate : Concatenate  NumInputs=4  Mode=Multidimensional array
  Matrix Concatenate1 : Concatenate  NumInputs=3  Mode=Multidimensional array
  Product : Product
  Scope : Scope
      settings: ActiveDisplayYMinimum=-0.00016  ActiveDisplayYMaximum=0.00015
  Selector : Selector  NumberOfDimensions=2  InputPortWidth=3  IndexOptions=Index vector (dialog),Select all  Indices=1,1  OutputSizes=1,1
  Selector1 : Selector  NumberOfDimensions=2  InputPortWidth=3  IndexOptions=Index vector (dialog),Select all  Indices=2,1  OutputSizes=1,1
  Selector10 : Selector  NumberOfDimensions=2  InputPortWidth=3  IndexOptions=Index vector (dialog),Select all  Indices=2,1  OutputSizes=1,1
  Selector11 : Selector  NumberOfDimensions=2  InputPortWidth=3  IndexOptions=Index vector (dialog),Select all  Indices=4,1  OutputSizes=1,1
  Selector2 : Selector  NumberOfDimensions=2  InputPortWidth=3  IndexOptions=Index vector (dialog),Select all  Indices=3,1  OutputSizes=1,1
  Selector3 : Selector  NumberOfDimensions=2  InputPortWidth=3  IndexOptions=Index vector (dialog),Select all  Indices=4,1  OutputSizes=1,1
  Selector4 : Selector  NumberOfDimensions=2  InputPortWidth=3  IndexOptions=Index vector (dialog),Select all  Indices=5,1  OutputSizes=1,1
  Selector5 : Selector  NumberOfDimensions=2  InputPortWidth=3  IndexOptions=Index vector (dialog),Select all  Indices=6,1  OutputSizes=1,1
  Selector6 : Selector  NumberOfDimensions=2  InputPortWidth=3  IndexOptions=Index vector (dialog),Select all  Indices=1:4,1  OutputSizes=1,1
  Selector7 : Selector  NumberOfDimensions=2  InputPortWidth=3  IndexOptions=Index vector (dialog),Select all  Indices=1,1  OutputSizes=1,1
  Selector8 : Selector  NumberOfDimensions=2  InputPortWidth=3  IndexOptions=Index vector (dialog),Select all  Indices=3,1  OutputSizes=1,1
  Selector9 : Selector  NumberOfDimensions=2  InputPortWidth=3  IndexOptions=Index vector (dialog),Select all  Indices=1,1  OutputSizes=1,1
  Sum{,1..3,5} (5 alike) : Sum  Inputs=|++
  Sum4 : Sum  Inputs=|-+
  Sum6 : Sum  Inputs=|+-
  Switch : Switch  Criteria=u2 > Threshold  SaturateOnIntegerOverflow=off  InputSameDT=off
  Transpose{,1..11} (12 alike) : Math  Operator=transpose
  start_SC1 : InportShadow  Port=2
  secondary_refs : Outport
  wires:
  Selector3/1 -> Transpose3/1  "Q"
  Selector/1 -> Transpose/1  "f"
  Selector1/1 -> Transpose1/1  "P"
  Selector2/1 -> Transpose2/1  "v"
  Gain/1 -> Sum/1
  Sum/1 -> Transpose4/1
  Gain1/1 -> Sum/2
  Gain2/1 -> Sum1/1
  Gain3/1 -> Sum1/2
  Sum1/1 -> Transpose5/1
  Gain4/1 -> Sum2/1
  Gain5/1 -> Sum2/2
  Gain6/1 -> Sum3/2
  Sum2/1 -> Transpose6/1
  Sum3/1 -> Transpose7/1
  Gain7/1 -> Sum3/1
  Transpose/1 -> Gain/1
  Transpose1/1 -> Gain2/1
  Transpose2/1 -> Gain4/1
  Transpose3/1 -> Gain7/1
  Transpose4/1 -> Matrix Concatenate/1
  Transpose6/1 -> Matrix Concatenate/3
  Transpose7/1 -> Matrix Concatenate/4
  Selector8/1 -> Transpose10/1
  Selector4/1 -> Matrix Concatenate1/2
  start_SC/1 -> Switch/2
  Switch/1 -> secondary_refs/1
  tertiary_refs/1 -> Switch/3, Sum5/2, Selector5/1, Selector4/1, Sum4/1
  Transpose5/1 -> Matrix Concatenate/2
  elec/1 -> Sum4/2
  Selector5/1 -> Matrix Concatenate1/3
  Selector9/1 -> Transpose8/1
  Selector10/1 -> Transpose9/1
  Selector11/1 -> Transpose11/1
  Matrix Concatenate1/1 -> Sum5/1
  Sum5/1 -> Switch/1
  Transpose8/1 -> Gain1/1
  Transpose9/1 -> Gain3/1
  Transpose10/1 -> Gain5/1
  Transpose11/1 -> Gain6/1
  Sum4/1 -> Selector6/1, Gain9/1, Selector2/1, Selector3/1, Selector1/1, Selector/1
  Integrator/1 -> Matrix Concatenate1/1
  Matrix Concatenate/1 -> Sum6/1
  Selector6/1 -> Gain10/1
  Gain9/1 -> Selector11/1, Selector8/1, Selector10/1, Selector9/1
  Product/1 -> Integrator/1
  Sum6/1 -> Selector7/1, Gain8/1
  Selector7/1 -> Scope/1
  Gain8/1 -> Product/1
  start_SC1/1 -> Product/2
  Gain10/1 -> Sum6/2

== system VFlexP/Grid/Secondary Control/Matrices with delay ==
  tertiary_refs : Inport
  elec : Inport  Port=2
  start_SC : Inport  Port=3
  Assignment : Assignment  NumberOfDimensions=2  DiagnosticForDimensions=Warning  IndexOptions=Index vector (dialog),Assign all  Indices=1,1  OutputSizes=1,1
  Assignment1 : Assignment  NumberOfDimensions=2  DiagnosticForDimensions=Warning  IndexOptions=Index vector (dialog),Assign all  Indices=2,1  OutputSizes=1,1
  For Each Subsystem : Subsystem  TreatAsAtomicUnit=on  mask{delayM=delayM, A_f_sc=A_f_sc}
  For Each Subsystem1 : Subsystem  TreatAsAtomicUnit=on  mask{delayM=delayM, A_P_sc=A_P_sc}
  For Each Subsystem2 : Subsystem  TreatAsAtomicUnit=on  mask{delayM=delayM, A_v_sc=A_v_sc}
  For Each Subsystem3 : Subsystem  TreatAsAtomicUnit=on  mask{delayM=delayM, A_Q_sc=A_Q_sc}
  Gain : Gain  Gain=-1
  Gain1 : Gain  Gain=g_f_sc'
  Gain2 : Gain  Gain=[sum(A_f_sc, 2)'; sum(A_P_sc, 2)'; sum(A_v_sc, 2)'; sum(A_Q_sc, 2)']
  Gain3 : Gain  Gain=g_P_sc'
  Gain5 : Gain  Gain=g_v_sc'
  Gain6 : Gain  Gain=g_Q_sc'
  Gain8 : Gain
  Integrator : Integrator
  Matrix Concatenate : Concatenate  NumInputs=4  Mode=Multidimensional array
  Matrix Concatenate1 : Concatenate  NumInputs=3  Mode=Multidimensional array
  Selector : Selector  NumberOfDimensions=2  InputPortWidth=3  IndexOptions=Index vector (dialog),Select all  Indices=1,1  OutputSizes=1,1
  Selector1 : Selector  NumberOfDimensions=2  InputPortWidth=3  IndexOptions=Index vector (dialog),Select all  Indices=2,1  OutputSizes=1,1
  Selector10 : Selector  NumberOfDimensions=2  InputPortWidth=3  IndexOptions=Index vector (dialog),Select all  Indices=2,1  OutputSizes=1,1
  Selector11 : Selector  NumberOfDimensions=2  InputPortWidth=3  IndexOptions=Index vector (dialog),Select all  Indices=4,1  OutputSizes=1,1
  Selector12 : Selector  NumberOfDimensions=2  InputPortWidth=3  IndexOptions=Index vector (dialog),Select all  Indices=2,1  OutputSizes=1,1
  Selector2 : Selector  NumberOfDimensions=2  InputPortWidth=3  IndexOptions=Index vector (dialog),Select all  Indices=3,1  OutputSizes=1,1
  Selector3 : Selector  NumberOfDimensions=2  InputPortWidth=3  IndexOptions=Index vector (dialog),Select all  Indices=4,1  OutputSizes=1,1
  Selector4 : Selector  NumberOfDimensions=2  InputPortWidth=3  IndexOptions=Index vector (dialog),Select all  Indices=6,1  OutputSizes=1,1
  Selector5 : Selector  NumberOfDimensions=2  InputPortWidth=3  IndexOptions=Index vector (dialog),Select all  Indices=5,1  OutputSizes=1,1
  Selector6 : Selector  NumberOfDimensions=2  InputPortWidth=3  IndexOptions=Index vector (dialog),Select all  Indices=1:4,1  OutputSizes=1,1
  Selector7 : Selector  NumberOfDimensions=2  InputPortWidth=3  IndexOptions=Index vector (dialog),Select all  Indices=1,1  OutputSizes=1,1
  Selector8 : Selector  NumberOfDimensions=2  InputPortWidth=3  IndexOptions=Index vector (dialog),Select all  Indices=3,1  OutputSizes=1,1
  Selector9 : Selector  NumberOfDimensions=2  InputPortWidth=3  IndexOptions=Index vector (dialog),Select all  Indices=1,1  OutputSizes=1,1
  Sum{,1..3,5,7..8} (7 alike) : Sum  Inputs=|++
  Sum of Elements{,1..3} (4 alike) : Sum  Inputs=+  CollapseMode=Specified dimension  CollapseDim=2
  Sum4 : Sum  Inputs=|-+
  Sum6 : Sum  Inputs=|+-
  Switch : Switch  Criteria=u2 > Threshold  SaturateOnIntegerOverflow=off  InputSameDT=off
  Transpose{,1..11} (12 alike) : Math  Operator=transpose
  Zero : Constant  Value=zeros(1, length(buses_lf))  VectorParams1D=off  OutDataTypeStr=Inherit: Inherit via back propagation
  secondary_refs : Outport
  wires:
  Selector3/1 -> Transpose3/1  "Q"
  Selector/1 -> Transpose/1  "f"
  Selector1/1 -> Transpose1/1  "P"
  Selector2/1 -> Transpose2/1  "v"
  Selector4/1 -> Matrix Concatenate1/3
  Sum/1 -> Transpose4/1
  Gain1/1 -> Sum/2
  Gain3/1 -> Sum1/2
  Sum1/1 -> Transpose5/1
  Sum of Elements2/1 -> Sum2/1
  Gain5/1 -> Sum2/2
  Gain6/1 -> Sum3/2
  Sum2/1 -> Transpose6/1
  Sum3/1 -> Transpose7/1
  Sum of Elements3/1 -> Sum3/1
  Transpose/1 -> For Each Subsystem/1(In1)
  Transpose1/1 -> For Each Subsystem1/1(In1)
  Transpose2/1 -> For Each Subsystem2/1(In1)
  Transpose3/1 -> For Each Subsystem3/1(In1)
  Transpose4/1 -> Matrix Concatenate/1
  Transpose6/1 -> Matrix Concatenate/3
  Transpose7/1 -> Matrix Concatenate/4
  For Each Subsystem/1(Out1) -> Sum of Elements/1
  For Each Subsystem1/1(Out1) -> Sum of Elements1/1
  For Each Subsystem2/1(Out1) -> Sum of Elements2/1
  For Each Subsystem3/1(Out1) -> Sum of Elements3/1
  Switch/1 -> secondary_refs/1
  Transpose5/1 -> Matrix Concatenate/2
  tertiary_refs/1 -> Sum5/2, Switch/3, Selector4/1, Selector5/1, Sum4/1
  elec/1 -> Sum4/2
  Matrix Concatenate1/1 -> Sum5/1
  Sum5/1 -> Switch/1
  Selector10/1 -> Transpose9/1
  Selector8/1 -> Transpose10/1
  Selector11/1 -> Transpose11/1
  Sum4/1 -> Gain/1, Selector2/1, Selector6/1, Selector3/1, Selector1/1, Selector/1
  Selector9/1 -> Transpose8/1
  Sum6/1 -> Gain8/1
  Matrix Concatenate/1 -> Sum6/1
  Selector6/1 -> Gain2/1
  start_SC/1 -> Switch/2
  Transpose8/1 -> Gain1/1
  Transpose9/1 -> Gain3/1
  Transpose10/1 -> Gain5/1
  Transpose11/1 -> Gain6/1
  Gain/1 -> Selector11/1, Selector8/1, Selector10/1, Selector9/1
  Integrator/1 -> Matrix Concatenate1/1
  Gain8/1 -> Integrator/1
  Selector5/1 -> Matrix Concatenate1/2
  Gain2/1 -> Selector7/1, Selector12/1, Assignment/1
  Zero/1 -> Assignment/2
  Assignment/1 -> Assignment1/1
  Selector7/1 -> Sum7/1
  Selector12/1 -> Sum7/2
  Sum7/1 -> Assignment1/2
  Assignment1/1 -> Sum6/2
  Sum of Elements/1 -> Sum8/1
  Sum8/1 -> Sum1/1
  Sum of Elements1/1 -> Sum8/2
